simulink model "f16_8"  (R2019a)
settings: Solver=VariableStepAuto  StartTime=0.0  StopTime=150  RelTol=1e-3  AbsTol=1e-6
libraries: simulink_extras x7
(part 1 of 2)
settings Model: ExtModeTrigMode=oneshot  ExtModeArmWhenConnect=off  OrderedModelArguments=off  Creator=aemhl  LastModifiedBy=dn15825
settings SolverCC: AutoScaleAbsTol=off
settings DataIOCC: SaveFormat=Array  SignalLoggingSaveFormat=ModelDataLogs  ReturnWorkspaceOutputs=off
settings OptimizationCC: BlockReduction=off  BooleanDataType=off
settings DebuggingCC: SaveWithParameterizedLinksMsg=none  UnderspecifiedInitializationDetection=Classic  MergeDetectMultiDrivingBlocksExec=none  SignalResolutionControl=TryResolveAllWithWarning  MultiTaskDSMMsg=warning  MultiTaskCondExecSysMsg=none  InitInArrayFormatMsg=none  SFUnexpectedBacktrackingDiag=warning  SFNoUnconditionalDefaultTransitionDiag=warning  SFExecutionAtInitializationDiag=none  ArithmeticOperatorsInVariantConditions=warning
settings HardwareCC: ProdBitPerPointer=32  ProdBitPerSizeT=32  ProdBitPerPtrDiffT=32  ProdLargestAtomicFloat=None  ProdIntDivRoundTo=Undefined  ProdEndianess=Unspecified  ProdWordSize=32  ProdHWDeviceType=32-bit Generic  TargetBitPerPointer=64  TargetBitPerSizeT=64  TargetBitPerPtrDiffT=64  TargetLongLongMode=on  TargetIntDivRoundTo=Zero  TargetEndianess=LittleEndian  TargetWordSize=64  TargetHWDeviceType=MATLAB Host  ProdEqTarget=off
settings ModelReferenceCC: PropagateSignalLabelsOutOfModel=off
settings SFSimCC: SimUseLocalCustomCode=off
settings RTWCC: SystemTargetFile=rsim.tlc  TemplateMakefile=rsim_auto_vcx64.tmf  Description=Rapid Simulation Target  GenerateReport=on  RTWUseLocalCustomCode=off  LaunchReport=on  RTWCompilerOptimization=on
settings CodeAppCC: StateflowObjectComments=on
settings TargetCC: ParMdlRefBuildCompliant=on  ConcurrentExecutionCompliant=on  GeneratePreprocessorConditionals=Use local settings  MatFileLogging=on  PreserveStateflowLocalDataDimensions=off
settings ConfigComp: CovMetricSettings=dw  CovHtmlReporting=on  CovSaveCumulativeToWorkspaceVar=on  CovSaveSingleToWorkspaceVar=on  CovExternalEMLEnable=off  CovSFcnEnable=off

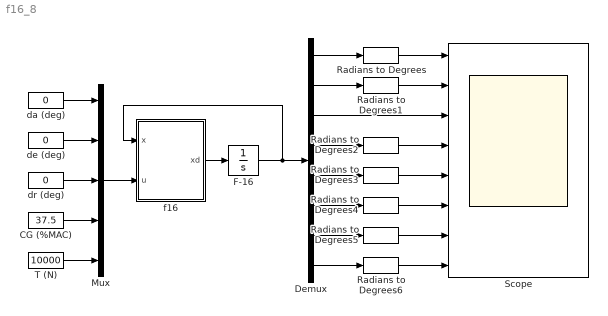
== system f16_8 ==
  CG (%MAC) : Constant  Value=37.5
  Demux : Demux  Outputs=8
  F-16 : Integrator  InitialCondition=[1.01392670620385;0;79.6036079039396;0;0;0;0;0.162105481242851]
  Mux : Mux  Inputs=5
  Radians to Degrees{,1..6} (7 alike) : simulink_extras/Transformations/Radians to Degrees
  Scope : Scope  NumInputPorts=8
  T (N) : Constant  Value=10000
  da (deg) : Constant  Value=0
  de (deg) : Constant  Value=0
  dr (deg) : Constant  Value=0
  f16 : MATLAB Function  TreatAsAtomicUnit=on
  wires:
  F-16/1 -> f16/1(x), Demux/1
  f16/1(xd) -> F-16/1
  Mux/1 -> f16/2(u)
  de (deg)/1 -> Mux/2
  CG (%MAC)/1 -> Mux/4
  T (N)/1 -> Mux/5
  da (deg)/1 -> Mux/1
  dr (deg)/1 -> Mux/3
  Demux/1 -> Radians to Degrees/1
  Demux/2 -> Radians to Degrees1/1
  Demux/3 -> Scope/3
  Demux/4 -> Radians to Degrees2/1
  Demux/5 -> Radians to Degrees3/1
  Demux/6 -> Radians to Degrees4/1
  Demux/7 -> Radians to Degrees5/1
  Demux/8 -> Radians to Degrees6/1
  Radians to Degrees1/1 -> Scope/2
  Radians to Degrees2/1 -> Scope/4
  Radians to Degrees3/1 -> Scope/5
  Radians to Degrees4/1 -> Scope/6
  Radians to Degrees5/1 -> Scope/7
  Radians to Degrees6/1 -> Scope/8
  Radians to Degrees/1 -> Scope/1
